simulink model "układZeroweWarunki"  (R2014a)
settings: Solver=ode45  StartTime=0.0  StopTime=10.0  MaxStep=0.01  RelTol=1e-3
values from neighbouring files (symbols this model uses):
  A = [-100 0 0 ... (first row only)    [zad1.m]
  B = [1000 ... (first row only)    [zad1.m]
  C = [0 0 0.4]    [zad1.m]
  G = [-990720; 10957.5; -77.5]    [zad1.m]
settings Model: Creator=Szwank  LastModifiedBy=Szwank

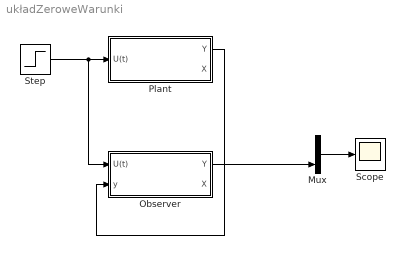
== system układZeroweWarunki ==
  Mux : Mux  Inputs=2
  "Observer " : Subsystem
  Plant : Subsystem
  Scope : Scope
  Step : Step  SampleTime=0
  wires:
  Step/1 -> "Observer "/1(U(t)), Plant/1(U(t))
  Plant/1(Y) -> "Observer "/2("y ")
  "Observer "/1(Y) -> Mux/2
  Mux/1 -> Scope/1

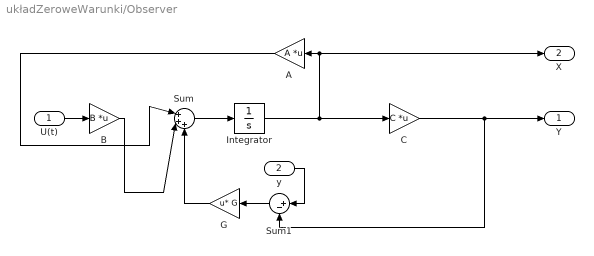
== system układZeroweWarunki/Observer  ==
  U(t) : Inport
  "y " : Inport  Port=2
  A : Gain  Gain=A  Multiplication=Matrix(K*u)
  B : Gain  Gain=B  Multiplication=Matrix(K*u)
  C : Gain  Gain=C  Multiplication=Matrix(K*u)
  G : Gain  Gain=G  Multiplication=Matrix(u*K)
  Integrator : Integrator
  Sum : Sum  Inputs=|+++
  Sum1 : Sum  Inputs=|+-
  Y : Outport
  X : Outport  Port=2
  wires:
  A/1 -> Sum/1
  U(t)/1 -> B/1
  Integrator/1 -> C/1, X/1, A/1
  C/1 -> Sum1/2, Y/1
  B/1 -> Sum/2
  Sum/1 -> Integrator/1
  "y "/1 -> Sum1/1
  Sum1/1 -> G/1
  G/1 -> Sum/3

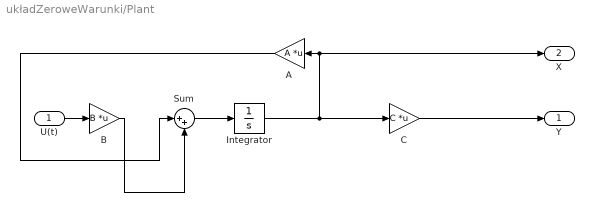
== system układZeroweWarunki/Plant ==
  U(t) : Inport
  A : Gain  Gain=A  Multiplication=Matrix(K*u)
  B : Gain  Gain=B  Multiplication=Matrix(K*u)
  C : Gain  Gain=C  Multiplication=Matrix(K*u)
  Integrator : Integrator
  Sum : Sum  Inputs=|++
  Y : Outport
  X : Outport  Port=2
  wires:
  A/1 -> Sum/1
  U(t)/1 -> B/1
  Integrator/1 -> C/1, X/1, A/1
  C/1 -> Y/1
  B/1 -> Sum/2
  Sum/1 -> Integrator/1
